simulink model "hyperbolic_tangent_sliding_mode"  (R2019b)
settings: Solver=VariableStepAuto  StartTime=0.0  StopTime=20  RelTol=1e-3
settings Model: Creator=Alien  LastModifiedBy=Alien
settings SolverCC: ZeroCrossAlgorithm=Adaptive
settings DebuggingCC: IgnoredZcDiagnostic=none

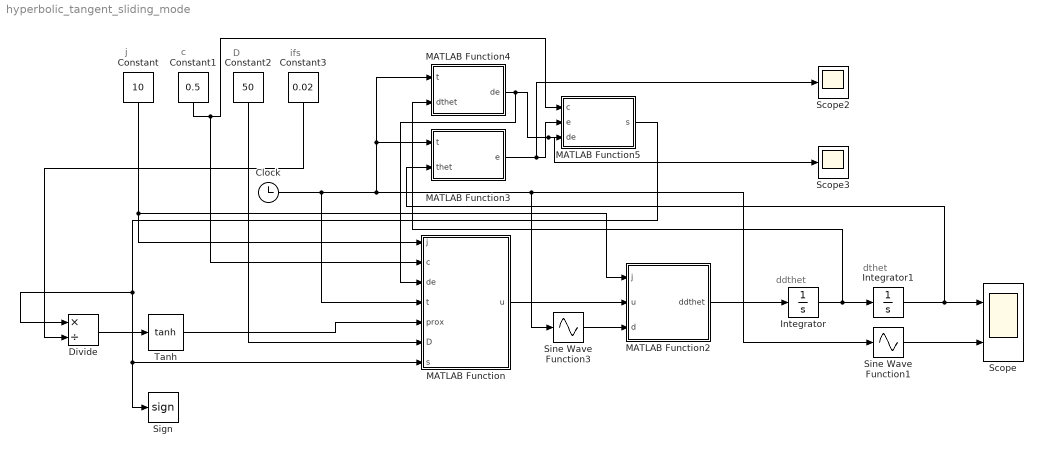
== system hyperbolic_tangent_sliding_mode ==
  note: ifs
  note: D
  note: c
  note: j
  note: ddthet
  note: dthet
  Clock : Clock
  Constant : Constant  Value=10
  Constant1 : Constant  Value=0.5
  Constant2 : Constant  Value=50
  Constant3 : Constant  Value=0.02
  Divide : Product  Inputs=*/
  Integrator : Integrator  InitialCondition=0.5
  Integrator1 : Integrator  InitialCondition=1
  MATLAB Function : MATLAB Function  TreatAsAtomicUnit=on
  MATLAB Function2 : MATLAB Function  TreatAsAtomicUnit=on
  MATLAB Function3 : MATLAB Function  TreatAsAtomicUnit=on
  MATLAB Function4 : MATLAB Function  TreatAsAtomicUnit=on
  MATLAB Function5 : MATLAB Function  TreatAsAtomicUnit=on
  Scope : Scope  NumInputPorts=2
  Scope2 : Scope
  Scope3 : Scope
  Sign : Signum
  Sine Wave Function1 : Sin  TimeSource=Use external signal  SampleTime=0
  Sine Wave Function3 : Sin  TimeSource=Use external signal  Amplitude=50  SampleTime=0
  Tanh : Trigonometry  Operator=tanh
  wires:
  Integrator/1 -> MATLAB Function4/2(dthet), Integrator1/1
  MATLAB Function2/1(ddthet) -> Integrator/1
  Constant1/1 -> MATLAB Function/2(c), MATLAB Function5/1(c)
  MATLAB Function4/1(de) -> MATLAB Function/3(de), Scope3/1, MATLAB Function5/3(de)
  MATLAB Function3/1(e) -> Scope2/1, MATLAB Function5/2(e)
  Integrator1/1 -> MATLAB Function3/2(thet), Scope/1
  Sine Wave Function1/1 -> Scope/2
  MATLAB Function5/1(s) -> MATLAB Function/7(s), Sign/1, Divide/1
  MATLAB Function/1(u) -> MATLAB Function2/2(u)
  Sine Wave Function3/1 -> MATLAB Function2/3(d)
  Divide/1 -> Tanh/1
  Constant3/1 -> Divide/2
  Clock/1 -> MATLAB Function/4(t), Sine Wave Function1/1, Sine Wave Function3/1, MATLAB Function4/1(t), MATLAB Function3/1(t)
  Constant2/1 -> MATLAB Function/6(D)
  Constant/1 -> MATLAB Function2/1(j), MATLAB Function/1(j)
  Tanh/1 -> MATLAB Function/5(prox)

== matlab function hyperbolic_tangent_sliding_mode/MATLAB Function ==
  data: j input; u output; c input; de input; t input; prox input; D input; s input
function u = fcn(j, c, de, t, prox, D, s)
nta = 0.5;
u = j*(-c*de - sin(t) - nta * s) - D*prox;

== matlab function hyperbolic_tangent_sliding_mode/MATLAB Function2 ==
  data: j input; ddthet output; u input; d input
function ddthet = fcn(j, u, d)
ddthet = 1/j*(u + d);

== matlab function hyperbolic_tangent_sliding_mode/MATLAB Function3 ==
  data: t input; e output; thet input
function e = fcn(t, thet)
e = thet - sin(t);

== matlab function hyperbolic_tangent_sliding_mode/MATLAB Function4 ==
  data: t input; de output; dthet input
function de = fcn(t, dthet)
de = dthet - cos(t);

== matlab function hyperbolic_tangent_sliding_mode/MATLAB Function5 ==
  data: c input; s output; e input; de input
function s = fcn(c, e, de)
s = c * e + de;
